simulink model "Model"  (R2024b)
settings: Solver=ode45  StartTime=0.0  StopTime=20  FixedStep=0.0005  MaxStep=InternalTs  RelTol=1e-3
InitFcn:
  | Design
values from neighbouring files (symbols this model uses):
  A = T \ A * T    [Design.m]
  Ao = A - L*C    [Design.m]
  B = T \ B    [Design.m]
  Bo = [B, L]    [Design.m]
  C = [1, 0, 0, 0]    [Design.m]
  D = 0    [Design.m]
  K = TmpK(2:end)    [Design.m]
  Ki = TmpK(1)    [Design.m]
  Nr = Nu + K * Nx    [Design.m]
  Ref = 50    [Design.m]
undefined symbols (not defined in the file or in its folder): DiscIntNeverNeededParam, InternalTs, RD, sens, t1
libraries: simulink_extras x6, simulink x2
settings Model: Creator=Banaan  LastModifiedBy=Banaan

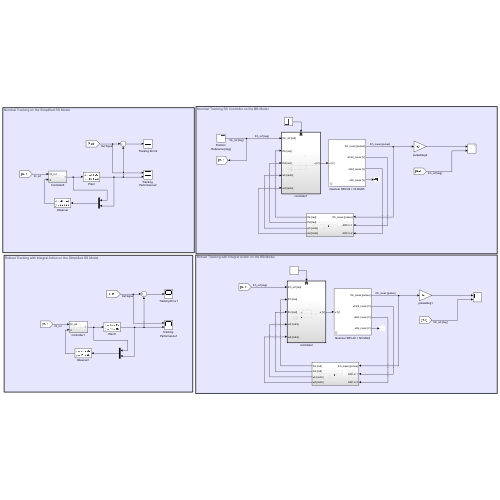
[thumbnail: Simulink's stored preview of the top-level diagram]
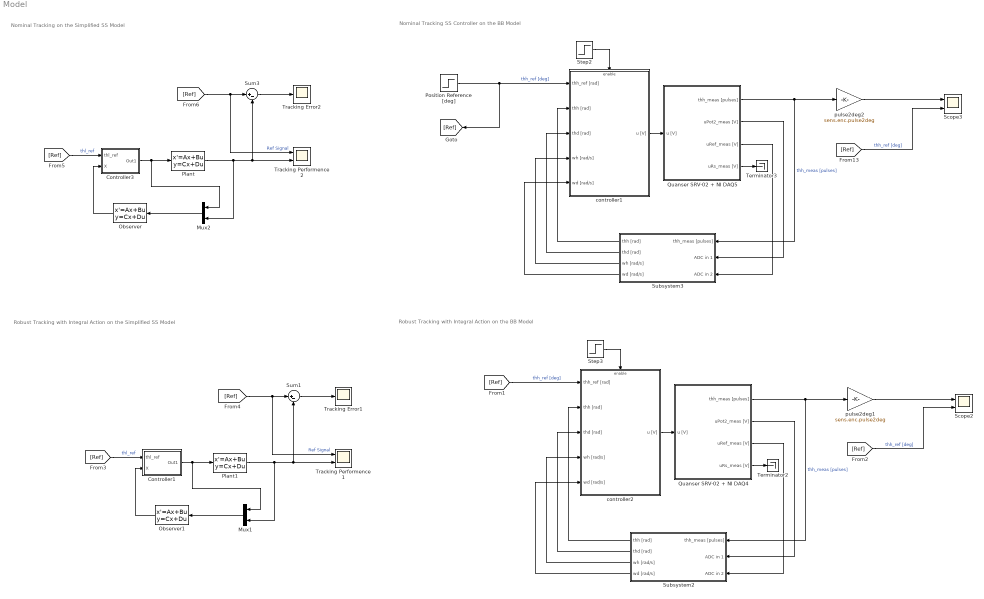
== system Model ==
  note: Robust Tracking with Integral Action on the BB Model
  note: Robust Tracking with Integral Action on the Simplified SS Model
  note: Nominal Tracking on the Simplified SS Model
  note: Nominal Tracking SS Controller on the BB Model
  Controller1 : Subsystem
  Controller3 : Subsystem
  Mux1 : Mux  Inputs=2
  Mux2 : Mux  Inputs=2
  Observer : StateSpace  A=Ao  B=Bo  C=eye(4)  D=zeros(4, 2)  InitialCondition=0
  Observer1 : StateSpace  A=Ao  B=Bo  C=eye(4)  D=zeros(4, 2)  InitialCondition=0
  Plant : StateSpace  A=A  B=B  C=C  D=D  InitialCondition=0
  Plant1 : StateSpace  A=A  B=B  C=C  D=D  InitialCondition=0
  Position Reference [deg] : Step  After=Ref  SampleTime=0
  Quanser SRV-02 + NI DAQ4 : Subsystem  mask(Quanser SRV-02 (with resonant load) + NI DAQ){Ts=0.001, fricType=Coulomb + viscous, lockShaft=off, beamInitPos=10}
      mask prompts: Ts "NI DAQ Sample Time:"; fricType "Friction model"; lockShaft "Lock motor shaft"; beamInitPos "Beam initial position [deg]:"
      mask help: Quanser SRV-02 (with resonant load) + NI DAQ model.
      mask init:
      | %%
      | % Riccardo Antonello (riccardo.antonello@unipd.it)
      | %
      | % April 28, 2020
      | %
      | % Dept. of Information Engineering, University of Padova
      | %
      | 
      | %%  Conversion gains
      | deg2rad = pi/180;                   %   [deg]   -> [rad]
      | rad2deg = 180/pi;                   %   [rad]   -> [deg]
      | 
      | 
      | %%  Sensors data
      | 
      | %   shunt resistor
      | sens.curr.Rs = 0.5;   
      | 
      | %   Hewlett-Packard HEDS-5540#A06 optical encoder
      | sens.enc.ppr = 500*4;                                                   %   pulses per rotation
      | sens.enc.pulse2deg = 360/sens.enc.ppr;                                  %   [pulses] -> [deg]
      | sens.enc.pulse2rad = 2*pi/sens.enc.ppr;                                 %   [pulses] -> [rad]
      | sens.enc.deg2pulse = sens.enc.ppr/360;                                  %   [deg] -> [pulses]
      | sens.enc.rad2pulse = sens.enc.ppr/2/pi;                                 %   [rad] -> [pulses]
      | 
      | %   potentiometer 2 (Spectrol 357-0-0-103) - installed on hub
      | sens.pot2.range.R      = 10e3;                                          %   ohmic value range 
      | sens.pot2.range.V      = 5;                                             %   voltage range
      | sens.pot2.range.th_deg = 340;                                           %   angle range [deg]
      | sens.pot2.range.th     = sens.pot2.range.th_deg * deg2rad;              %   angle range [rad]                           
      | sens.pot2.deg2V        = sens.pot2.range.V / sens.pot2.range.th_deg;    %   sensitivity [V/deg]
      | sens.pot2.rad2V        = sens.pot2.range.V / sens.pot2.range.th;        %   sensitivity [V/rad]
      | sens.pot2.V2deg        = 1/sens.pot2.deg2V;                             %   conversion gain [V] -> [deg]
      | sens.pot2.V2rad        = 1/sens.pot2.rad2V;                             %   conversion gain [V] -> [rad]
      | sens.pot2.noise.var    = 3.5e-7;                                        %   out noise variance [V^2]
      | 
      | 
      | %%  Data acquisition board (daq) data
      | 
      | %   NI PCI-6221 DAC data
      | daq.dac.bits = 16;                                  %   resolution (bits)
      | daq.dac.fs   = 10;                                  %   full scale 
      | daq.dac.q    = 2*daq.dac.fs/(2^daq.dac.bits-1);     %	quantization
      | 
      | %   NI PCI-6221 ADC data
      | daq.adc.bits = 16;                                  %   resolution (bits)
      | daq.adc.fs   = 10;                                  %   full scale (as set in SLDRT Analog Input block)
      | daq.adc.q    = 2*daq.adc.fs/(2^daq.adc.bits-1);     %   quantization   
      | 
      | 
      | %%  Set beam initial position
      | % SRV02Handle = find_system(gcb, ...
      | %     'LookUnderMasks', 'on', ...
      | %     'FindAll', 'on', ...
      | %     'FollowLinks', 'on', ...
      | %     'SearchDepth', '1', ...
      | %     'BlockType', 'ModelReference', ...
      | %     'Name', 'Quanser SRV-02');
      | %
      | % %get_param(SRV02Handle, 'InstanceParameters')
      | % InstanceParams = get_param(SRV02Handle, 'InstanceParameters');
      | % for k = 1:length(InstanceParams)
      | %     if strcmp(InstanceParams(k).Name, 'thb0')
      | %         if lockShaft
      | %             InstanceParams(k).Value = sprintf('%f', beamInitPos);
      | %         else
      | %             InstanceParams(k).Value = sprintf('%f', 0);    
      | %         end
      | %         set_param(SRV02Handle, 'InstanceParameters', InstanceParams);
      | %         break;
      | %     end
      | % end
      | 
      | if lockShaft
      |     thb0 = beamInitPos;
      | else
      |     thb0 = 0;    
      | end
      | 
      | 
      | %%  Mask initialization
      | if lockShaft
      |     
      |     %   find Inport handle
      |     InPortHandle = find_system(gcb, ...
      |         'LookUnderMasks', 'on', ...
      |         'FindAll', 'on', ...
      |         'FollowLinks', 'on', ...
      |         'SearchDepth', '1', ...
      |         'BlockType', 'Inport', ...
      |         'Name', 'u [V]');
      |     
      |     if ~isempty(InPortHandle)
      |     
      |         %   find DAC handle
      |         DACHandle = find_system(gcb, ...
      |             'LookUnderMasks', 'on', ...
      |             'FindAll', 'on', ...
      |             'FollowLinks', 'on', ...
      |             'SearchDepth', '1', ...
      |             'BlockType', 'SubSystem', ...
      |             'Name', 'DAC');  
      | 
      |         %   remove Inport output connection   
      |         InportConn = get_param(InPortHandle, 'PortConnectivity');
      |         delete_line(gcb, InportConn.Position);
      | 
      |         %   remove Inport block
      |         delete_block(InPortHandle);
      | 
      |         %   add Constant block
      |         ConstantHandle = add_block( ...
      |             'simulink/Sources/Constant', [gcb, '/u [V]'], ...
      |             'Position', [20   -37    50   -23], ...
      |             'Value', '0');
      | 
      |         %   connect Constant to DAC block
      |         DACPortHandles = get_param(DACHandle, 'PortHandles');
      |         ConstantPortHandles = get_param(ConstantHandle, 'PortHandles');
      |         add_line(gcb, ConstantPortHandles.Outport(1), DACPortHandles.Inport(1));
      |     
      |     end
      |     
      | else
      |     
      |     %   find Constant handle
      |     ConstantHandle = find_system(gcb, ...
      |         'LookUnderMasks', 'on', ...
      |         'FindAll', 'on', ...
      |         'FollowLinks', 'on', ...
      |         'SearchDepth', '1', ...
      |         'BlockType', 'Constant', ...
      |         'Name', 'u [V]');
      |     
      |     if ~isempty(ConstantHandle)
      |     
      |         %   find DAC handle
      |         DACHandle = find_system(gcb, ...
      |             'LookUnderMasks', 'on', ...
      |             'FindAll', 'on', ...
      |             'FollowLinks', 'on', ...
      |             'SearchDepth', '1', ...
      |             'BlockType', 'SubSystem', ...
      |             'Name', 'DAC');  
      |  
      |         %   remove Constant output connection   
      |         ConstantConn = get_param(ConstantHandle, 'PortConnectivity');
      |         delete_line(gcb, ConstantConn.Position);
      | 
      |         %   remove Inport block
      |         delete_block(ConstantHandle);   
      | 
      |         %   add Inport block
      |         InportHandle = add_block( ...
      |             'simulink/Sources/In1', [gcb, '/u [V]'], ...
      |             'Position', [20   -37    50   -23], ...
      |             'Port', '1');
      | 
      |         %   connect Constant to DAC block
      |         DACPortHandles = get_param(DACHandle, 'PortHandles');
      |         InportPortHandles = get_param(InportHandle, 'PortHandles');
      |         add_line(gcb, InportPortHandles.Outport(1), DACPortHandles.Inport(1));
      |     
      |      end
      |     
      | end
      mask Help:
      | Riccardo Antonello (antonello@dei.unipd.it)
      | 
      | April 28, 2020
      | 
      | Dept. of Information Engineering, University of Padova
      mask TypeOptions fricType: Coulomb + viscous | Karnopp
      mask Callback lockShaft:
      | %   get status of check box
      | lockShaft = get_param(gcb, 'lockShaft');
      | 
      | %   get current value of MaskVisibilities property
      | maskVisibilities = get_param(gcb, 'MaskVisibilities');
      | 
      | %   set visibility of the dialog box element
      | if strcmp(lockShaft, 'on')
      |     maskVisibilities{4} = 'on';
      | else
      |     maskVisibilities{4} = 'off';
      | end
      | 
      | % Set the 'MaskVisibilities' property for each parameter in mask
      | set_param( gcb, 'MaskVisibilities', maskVisibilities);
  Quanser SRV-02 + NI DAQ5 : Subsystem  mask(Quanser SRV-02 (with resonant load) + NI DAQ){Ts=0.001, fricType=Coulomb + viscous, lockShaft=off, beamInitPos=10}
      mask prompts: Ts "NI DAQ Sample Time:"; fricType "Friction model"; lockShaft "Lock motor shaft"; beamInitPos "Beam initial position [deg]:"
      mask help: Quanser SRV-02 (with resonant load) + NI DAQ model.
      mask init: same as Model/Quanser SRV-02 + NI DAQ4
      mask Help:
      | Riccardo Antonello (antonello@dei.unipd.it)
      | 
      | April 28, 2020
      | 
      | Dept. of Information Engineering, University of Padova
      mask TypeOptions fricType: Coulomb + viscous | Karnopp
      mask Callback lockShaft:
      | %   get status of check box
      | lockShaft = get_param(gcb, 'lockShaft');
      | 
      | %   get current value of MaskVisibilities property
      | maskVisibilities = get_param(gcb, 'MaskVisibilities');
      | 
      | %   set visibility of the dialog box element
      | if strcmp(lockShaft, 'on')
      |     maskVisibilities{4} = 'on';
      | else
      |     maskVisibilities{4} = 'off';
      | end
      | 
      | % Set the 'MaskVisibilities' property for each parameter in mask
      | set_param( gcb, 'MaskVisibilities', maskVisibilities);
  Scope2 : Scope  NumInputPorts=2
  Scope3 : Scope  NumInputPorts=2
  Step2 : Step  Time=t1 + 0.01  SampleTime=0
  Step3 : Step  Time=t1 + 0.01  SampleTime=0
  Subsystem2 : Subsystem
  Subsystem3 : Subsystem
  Sum1 : Sum  Inputs=|+-
  Sum3 : Sum  Inputs=|+-
  Terminator2 : Terminator
  Terminator3 : Terminator
  Tracking Performence1 : Scope  NumInputPorts=2
  Tracking Performence2 : Scope  NumInputPorts=2
  Tracking Error1 : Scope
  Tracking Error2 : Scope
  controller1 : Subsystem
  controller2 : Subsystem
  pulse2deg1 : Gain  Gain=sens.enc.pulse2deg
  pulse2deg2 : Gain  Gain=sens.enc.pulse2deg
  wires:
  [Ref] -> Tracking Performence2/1, Sum3/1  "Ref Signal"
  Sum3/1 -> Tracking Error2/1
  Plant/1 -> Tracking Performence2/2, Sum3/2, Mux2/2
  Mux2/1 -> Observer/1
  [Ref] -> Scope3/2  "thh_ref [deg]"
  pulse2deg2/1 -> Scope3/1
  Subsystem3/4(wd [rad/s]) -> controller1/5(wd [rad/s])
  Subsystem3/3(wh [rad/s]) -> controller1/4(wh [rad/s])
  Subsystem3/2(thd [rad]) -> controller1/3(thd [rad])
  Subsystem3/1(thh [rad]) -> controller1/2(thh [rad])
  Quanser SRV-02 + NI DAQ5/3(uRef_meas [V]) -> Subsystem3/3(ADC in 2)
  Quanser SRV-02 + NI DAQ5/2(uPot2_meas [V]) -> Subsystem3/2(ADC in 1)
  Quanser SRV-02 + NI DAQ5/1(thh_meas [pulses]) -> Subsystem3/1(thh_meas [pulses]), pulse2deg2/1  "thh_meas [pulses]"
  controller1/1(u [V]) -> Quanser SRV-02 + NI DAQ5/1(u [V])
  Step2/1 -> controller1/Enable
  Quanser SRV-02 + NI DAQ5/4(uRs_meas [V]) -> Terminator3/1
  Position Reference [deg]/1 -> controller1/1(thh_ref [rad]), [Ref]  "thh_ref [deg]"
  Controller3/1(Out1) -> Plant/1, Mux2/1
  [Ref] -> Controller3/1(thl_ref)  "thl_ref"
  Observer/1 -> Controller3/2(X)
  [Ref] -> controller2/1(thh_ref [rad])  "thh_ref [deg]"
  Quanser SRV-02 + NI DAQ4/4(uRs_meas [V]) -> Terminator2/1
  Step3/1 -> controller2/Enable
  controller2/1(u [V]) -> Quanser SRV-02 + NI DAQ4/1(u [V])
  Quanser SRV-02 + NI DAQ4/1(thh_meas [pulses]) -> pulse2deg1/1, Subsystem2/1(thh_meas [pulses])  "thh_meas [pulses]"
  Quanser SRV-02 + NI DAQ4/2(uPot2_meas [V]) -> Subsystem2/2(ADC in 1)
  Quanser SRV-02 + NI DAQ4/3(uRef_meas [V]) -> Subsystem2/3(ADC in 2)
  Subsystem2/1(thh [rad]) -> controller2/2(thh [rad])
  Subsystem2/2(thd [rad]) -> controller2/3(thd [rad])
  Subsystem2/3(wh [rad/s]) -> controller2/4(wh [rad/s])
  Subsystem2/4(wd [rad/s]) -> controller2/5(wd [rad/s])
  pulse2deg1/1 -> Scope2/1
  [Ref] -> Scope2/2  "thh_ref [deg]"
  Observer1/1 -> Controller1/2(X)
  [Ref] -> Controller1/1(thl_ref)  "thl_ref"
  Controller1/1(Out1) -> Mux1/1, Plant1/1
  Mux1/1 -> Observer1/1
  Plant1/1 -> Mux1/2, Sum1/2, Tracking Performence1/2
  Sum1/1 -> Tracking Error1/1
  [Ref] -> Sum1/1, Tracking Performence1/1  "Ref Signal"

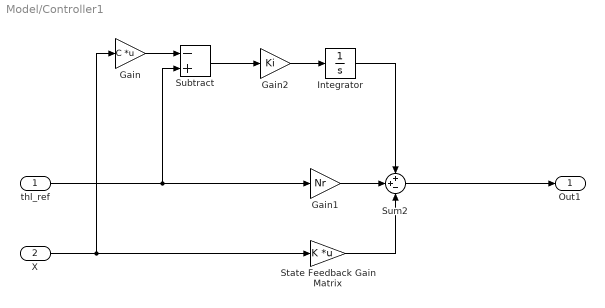
== system Model/Controller1 ==
  thl_ref : Inport
  X : Inport  Port=2
  Gain : Gain  Gain=C  Multiplication=Matrix(K*u)
  Gain1 : Gain  Gain=Nr
  Gain2 : Gain  Gain=Ki
  Integrator : Integrator
  State Feedback Gain Matrix : Gain  Gain=K  Multiplication=Matrix(K*u)
  Subtract : Sum  Inputs=-+
  Sum2 : Sum  Inputs=++-
  Out1 : Outport
  wires:
  Sum2/1 -> Out1/1
  X/1 -> Gain/1, State Feedback Gain Matrix/1
  Gain1/1 -> Sum2/2
  State Feedback Gain Matrix/1 -> Sum2/3
  Gain/1 -> Subtract/1
  thl_ref/1 -> Gain1/1, Subtract/2
  Subtract/1 -> Gain2/1
  Gain2/1 -> Integrator/1
  Integrator/1 -> Sum2/1

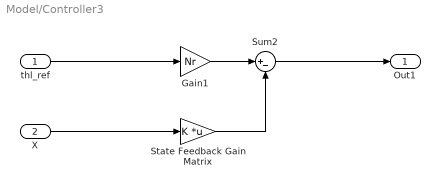
== system Model/Controller3 ==
  thl_ref : Inport
  X : Inport  Port=2
  Gain1 : Gain  Gain=Nr
  State Feedback Gain Matrix : Gain  Gain=K  Multiplication=Matrix(K*u)
  Sum2 : Sum  Inputs=|+-
  Out1 : Outport
  wires:
  State Feedback Gain Matrix/1 -> Sum2/2
  Gain1/1 -> Sum2/1
  X/1 -> State Feedback Gain Matrix/1
  thl_ref/1 -> Gain1/1
  Sum2/1 -> Out1/1

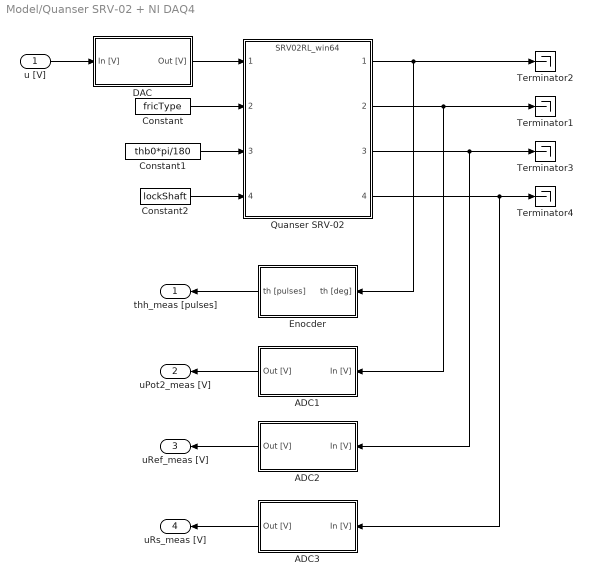
== system Model/Quanser SRV-02 + NI DAQ4 ==
  u [V] : Inport
  ADC1 : Subsystem
  ADC2 : Subsystem
  ADC3 : Subsystem
  Constant : Constant  Value=fricType
  Constant1 : Constant  Value=thb0*pi/180  SampleTime=Inf
  Constant2 : Constant  Value=lockShaft  SampleTime=Inf
  DAC : Subsystem
  Enocder : Subsystem
  Quanser SRV-02 : ModelReference  ModelNameDialog=SRV02RL_win64.slxp  ModelReferenceVersion=1.76  CopyOfModelProtected=on
  Terminator{1..4} (4 alike) : Terminator
  thh_meas [pulses] : Outport
  uPot2_meas [V] : Outport  Port=2
  uRef_meas [V] : Outport  Port=3
  uRs_meas [V] : Outport  Port=4
  wires:
  u [V]/1 -> DAC/1(In [V])
  ADC2/1(Out [V]) -> uRef_meas [V]/1
  Quanser SRV-02/4 -> Terminator4/1, ADC3/1(In [V])
  Constant2/1 -> Quanser SRV-02/4
  Constant1/1 -> Quanser SRV-02/3
  ADC1/1(Out [V]) -> uPot2_meas [V]/1
  Quanser SRV-02/3 -> Terminator3/1, ADC2/1(In [V])
  Constant/1 -> Quanser SRV-02/2
  Quanser SRV-02/1 -> Enocder/1(th [deg]), Terminator2/1
  Quanser SRV-02/2 -> Terminator1/1, ADC1/1(In [V])
  DAC/1(Out [V]) -> Quanser SRV-02/1
  ADC3/1(Out [V]) -> uRs_meas [V]/1
  Enocder/1(th [pulses]) -> thh_meas [pulses]/1

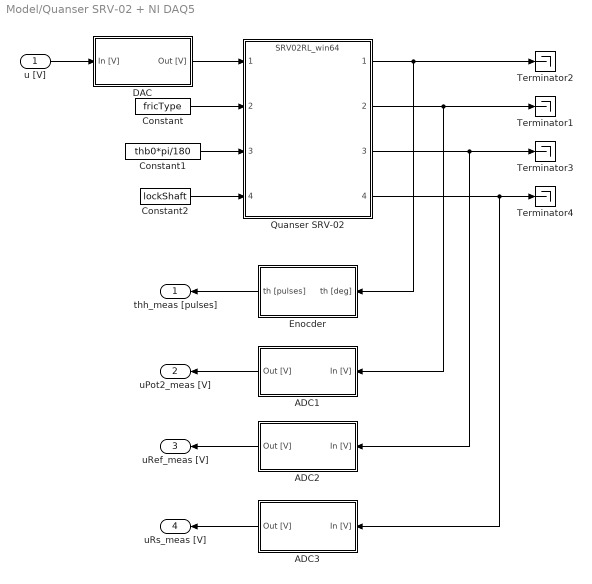
== system Model/Quanser SRV-02 + NI DAQ5 ==
  u [V] : Inport
  ADC1 : Subsystem
  ADC2 : Subsystem
  ADC3 : Subsystem
  Constant : Constant  Value=fricType
  Constant1 : Constant  Value=thb0*pi/180  SampleTime=Inf
  Constant2 : Constant  Value=lockShaft  SampleTime=Inf
  DAC : Subsystem
  Enocder : Subsystem
  Quanser SRV-02 : ModelReference  ModelNameDialog=SRV02RL_win64.slxp  ModelReferenceVersion=1.76  CopyOfModelProtected=on
  Terminator{1..4} (4 alike) : Terminator
  thh_meas [pulses] : Outport
  uPot2_meas [V] : Outport  Port=2
  uRef_meas [V] : Outport  Port=3
  uRs_meas [V] : Outport  Port=4
  wires:
  Enocder/1(th [pulses]) -> thh_meas [pulses]/1
  ADC3/1(Out [V]) -> uRs_meas [V]/1
  DAC/1(Out [V]) -> Quanser SRV-02/1
  Quanser SRV-02/2 -> ADC1/1(In [V]), Terminator1/1
  Quanser SRV-02/1 -> Terminator2/1, Enocder/1(th [deg])
  Constant/1 -> Quanser SRV-02/2
  Quanser SRV-02/3 -> ADC2/1(In [V]), Terminator3/1
  ADC1/1(Out [V]) -> uPot2_meas [V]/1
  Constant1/1 -> Quanser SRV-02/3
  Constant2/1 -> Quanser SRV-02/4
  Quanser SRV-02/4 -> ADC3/1(In [V]), Terminator4/1
  ADC2/1(Out [V]) -> uRef_meas [V]/1
  u [V]/1 -> DAC/1(In [V])

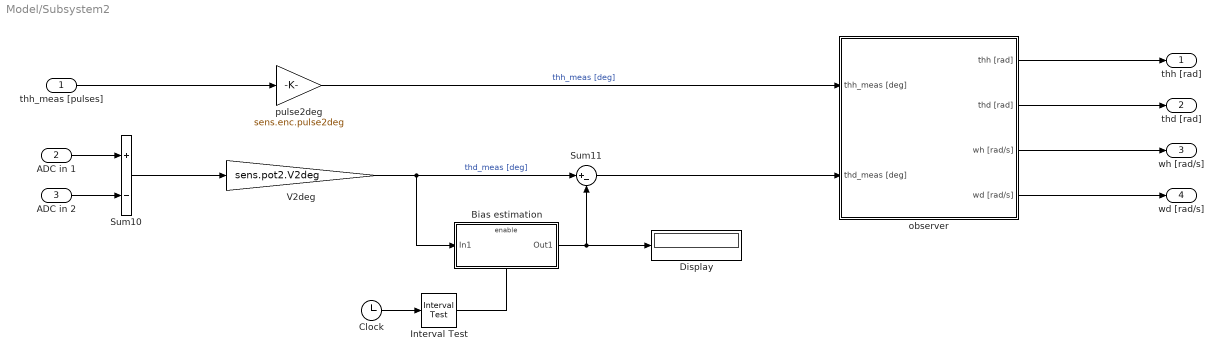
== system Model/Subsystem2 ==
  thh_meas [pulses] : Inport
  ADC in 1 : Inport  Port=2
  ADC in 2 : Inport  Port=3
  Bias estimation : Subsystem
  Clock : Clock
  Display : Display
  Interval Test : simulink/Logic and Bit Operations/Interval Test  IntervalClosedRight=on  uplimit=0.7  IntervalClosedLeft=on  lowlimit=0.2  OutDataTypeStr=boolean
  Sum10 : Sum  Inputs=+-
  Sum11 : Sum  Inputs=|+-
  V2deg : Gain  Gain=sens.pot2.V2deg
  observer : Subsystem
  pulse2deg : Gain  Gain=sens.enc.pulse2deg
  thh [rad] : Outport
  thd [rad] : Outport  Port=2
  wh [rad/s] : Outport  Port=3
  wd [rad/s] : Outport  Port=4
  wires:
  Bias estimation/1(Out1) -> Display/1, Sum11/2
  observer/1(thh [rad]) -> thh [rad]/1
  Interval Test/1 -> Bias estimation/Enable
  Sum10/1 -> V2deg/1
  thh_meas [pulses]/1 -> pulse2deg/1
  observer/4(wd [rad/s]) -> wd [rad/s]/1
  pulse2deg/1 -> observer/1(thh_meas [deg])  "thh_meas [deg]"
  ADC in 2/1 -> Sum10/2
  V2deg/1 -> Sum11/1, Bias estimation/1(In1)  "thd_meas [deg]"
  Sum11/1 -> observer/2(thd_meas [deg])
  Clock/1 -> Interval Test/1
  observer/2(thd [rad]) -> thd [rad]/1
  ADC in 1/1 -> Sum10/1
  observer/3(wh [rad/s]) -> wh [rad/s]/1

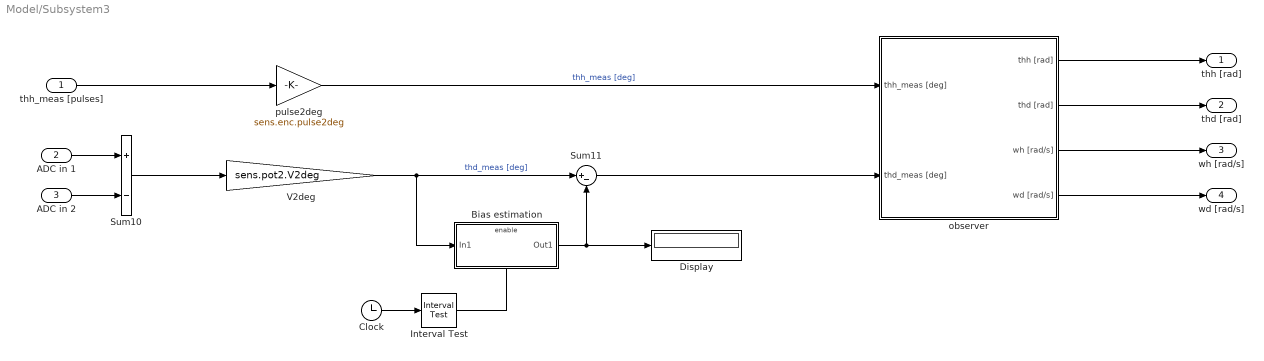
== system Model/Subsystem3 ==
  thh_meas [pulses] : Inport
  ADC in 1 : Inport  Port=2
  ADC in 2 : Inport  Port=3
  Bias estimation : Subsystem
  Clock : Clock
  Display : Display
  Interval Test : simulink/Logic and Bit Operations/Interval Test  IntervalClosedRight=on  uplimit=0.7  IntervalClosedLeft=on  lowlimit=0.2  OutDataTypeStr=boolean
  Sum10 : Sum  Inputs=+-
  Sum11 : Sum  Inputs=|+-
  V2deg : Gain  Gain=sens.pot2.V2deg
  observer : Subsystem
  pulse2deg : Gain  Gain=sens.enc.pulse2deg
  thh [rad] : Outport
  thd [rad] : Outport  Port=2
  wh [rad/s] : Outport  Port=3
  wd [rad/s] : Outport  Port=4
  wires:
  observer/3(wh [rad/s]) -> wh [rad/s]/1
  ADC in 1/1 -> Sum10/1
  observer/2(thd [rad]) -> thd [rad]/1
  Clock/1 -> Interval Test/1
  Sum11/1 -> observer/2(thd_meas [deg])
  V2deg/1 -> Bias estimation/1(In1), Sum11/1  "thd_meas [deg]"
  ADC in 2/1 -> Sum10/2
  pulse2deg/1 -> observer/1(thh_meas [deg])  "thh_meas [deg]"
  observer/4(wd [rad/s]) -> wd [rad/s]/1
  thh_meas [pulses]/1 -> pulse2deg/1
  Sum10/1 -> V2deg/1
  Interval Test/1 -> Bias estimation/Enable
  observer/1(thh [rad]) -> thh [rad]/1
  Bias estimation/1(Out1) -> Sum11/2, Display/1

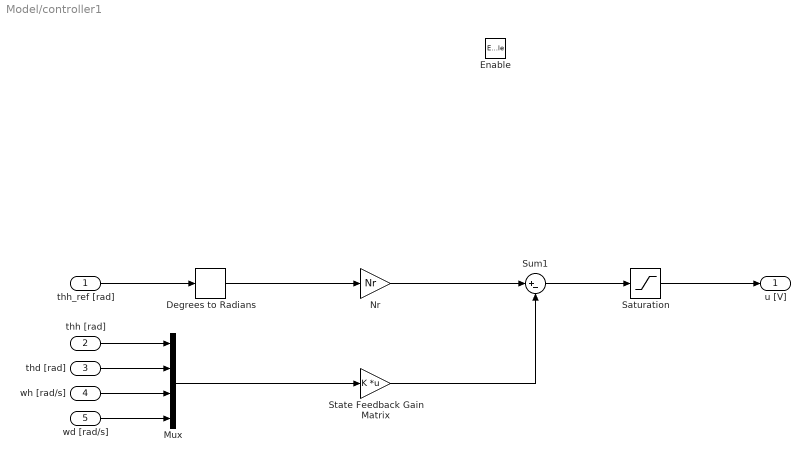
== system Model/controller1 ==
  thh_ref [rad] : Inport
  thh [rad] : Inport  Port=2
  thd [rad] : Inport  Port=3
  wh [rad/s] : Inport  Port=4
  wd [rad/s] : Inport  Port=5
  Enable : EnablePort
  Degrees to Radians : simulink_extras/Transformations/Degrees to Radians
  Mux : Mux
  Nr : Gain  Gain=Nr
  Saturation : Saturate  UpperLimit=10  LowerLimit=-10
  State Feedback Gain Matrix : Gain  Gain=K  Multiplication=Matrix(K*u)
  Sum1 : Sum  Inputs=|+-
  u [V] : Outport
  wires:
  Degrees to Radians/1 -> Nr/1
  Saturation/1 -> u [V]/1
  Mux/1 -> State Feedback Gain Matrix/1
  Nr/1 -> Sum1/1
  Sum1/1 -> Saturation/1
  wd [rad/s]/1 -> Mux/4
  wh [rad/s]/1 -> Mux/3
  thd [rad]/1 -> Mux/2
  thh [rad]/1 -> Mux/1
  State Feedback Gain Matrix/1 -> Sum1/2
  thh_ref [rad]/1 -> Degrees to Radians/1

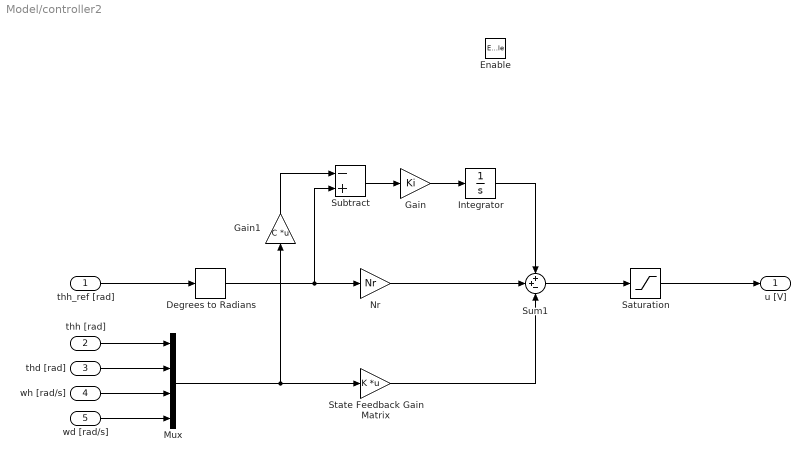
== system Model/controller2 ==
  thh_ref [rad] : Inport
  thh [rad] : Inport  Port=2
  thd [rad] : Inport  Port=3
  wh [rad/s] : Inport  Port=4
  wd [rad/s] : Inport  Port=5
  Enable : EnablePort
  Degrees to Radians : simulink_extras/Transformations/Degrees to Radians
  Gain : Gain  Gain=Ki
  Gain1 : Gain  Gain=C  Multiplication=Matrix(K*u)
  Integrator : Integrator
  Mux : Mux
  Nr : Gain  Gain=Nr
  Saturation : Saturate  UpperLimit=10  LowerLimit=-10
  State Feedback Gain Matrix : Gain  Gain=K  Multiplication=Matrix(K*u)
  Subtract : Sum  Inputs=-+
  Sum1 : Sum  Inputs=++-
  u [V] : Outport
  wires:
  thh_ref [rad]/1 -> Degrees to Radians/1
  State Feedback Gain Matrix/1 -> Sum1/3
  thh [rad]/1 -> Mux/1
  thd [rad]/1 -> Mux/2
  wh [rad/s]/1 -> Mux/3
  wd [rad/s]/1 -> Mux/4
  Sum1/1 -> Saturation/1
  Nr/1 -> Sum1/2
  Mux/1 -> State Feedback Gain Matrix/1, Gain1/1
  Saturation/1 -> u [V]/1
  Degrees to Radians/1 -> Subtract/2, Nr/1
  Gain/1 -> Integrator/1
  Subtract/1 -> Gain/1
  Integrator/1 -> Sum1/1
  Gain1/1 -> Subtract/1

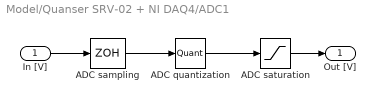
== system Model/Quanser SRV-02 + NI DAQ4/ADC1 ==
  In [V] : Inport
  ADC quantization : Quantizer  QuantizationInterval=daq.adc.q
  ADC sampling : ZeroOrderHold  SampleTime=Ts
  ADC saturation : Saturate  UpperLimit=daq.adc.fs  LowerLimit=-daq.adc.fs
  Out [V] : Outport
  wires:
  ADC quantization/1 -> ADC saturation/1
  In [V]/1 -> ADC sampling/1
  ADC sampling/1 -> ADC quantization/1
  ADC saturation/1 -> Out [V]/1

== system Model/Quanser SRV-02 + NI DAQ4/ADC2 ==
  In [V] : Inport
  ADC quantization : Quantizer  QuantizationInterval=daq.adc.q
  ADC sampling : ZeroOrderHold  SampleTime=Ts
  ADC saturation : Saturate  UpperLimit=daq.adc.fs  LowerLimit=-daq.adc.fs
  Out [V] : Outport
  wires:
  ADC saturation/1 -> Out [V]/1
  ADC sampling/1 -> ADC quantization/1
  In [V]/1 -> ADC sampling/1
  ADC quantization/1 -> ADC saturation/1

== system Model/Quanser SRV-02 + NI DAQ4/ADC3 ==
  In [V] : Inport
  Quantizer : Quantizer  QuantizationInterval=daq.adc.q
  Saturation : Saturate  UpperLimit=daq.adc.fs  LowerLimit=-daq.adc.fs
  Zero-Order Hold : ZeroOrderHold  SampleTime=Ts
  Out [V] : Outport
  wires:
  Zero-Order Hold/1 -> Quantizer/1
  Quantizer/1 -> Saturation/1
  In [V]/1 -> Zero-Order Hold/1
  Saturation/1 -> Out [V]/1

== system Model/Quanser SRV-02 + NI DAQ4/DAC ==
  In [V] : Inport
  Quantizer : Quantizer  QuantizationInterval=daq.dac.q
  Saturation : Saturate  UpperLimit=daq.dac.fs  LowerLimit=-daq.dac.fs
  Zero-Order Hold : ZeroOrderHold  SampleTime=Ts
  Out [V] : Outport
  wires:
  Saturation/1 -> Out [V]/1
  Zero-Order Hold/1 -> Quantizer/1
  In [V]/1 -> Zero-Order Hold/1
  Quantizer/1 -> Saturation/1

== system Model/Quanser SRV-02 + NI DAQ4/Enocder ==
  th [deg] : Inport
  Quantizer : Quantizer  QuantizationInterval=sens.enc.pulse2deg
  Zero-Order Hold : ZeroOrderHold  SampleTime=Ts
  deg2pulse : Gain  Gain=sens.enc.deg2pulse
  th [pulses] : Outport
  wires:
  deg2pulse/1 -> th [pulses]/1
  Zero-Order Hold/1 -> Quantizer/1
  th [deg]/1 -> Zero-Order Hold/1
  Quantizer/1 -> deg2pulse/1

== system Model/Quanser SRV-02 + NI DAQ5/ADC1 ==
  In [V] : Inport
  ADC quantization : Quantizer  QuantizationInterval=daq.adc.q
  ADC sampling : ZeroOrderHold  SampleTime=Ts
  ADC saturation : Saturate  UpperLimit=daq.adc.fs  LowerLimit=-daq.adc.fs
  Out [V] : Outport
  wires:
  ADC saturation/1 -> Out [V]/1
  ADC sampling/1 -> ADC quantization/1
  In [V]/1 -> ADC sampling/1
  ADC quantization/1 -> ADC saturation/1

== system Model/Quanser SRV-02 + NI DAQ5/ADC2 ==
  In [V] : Inport
  ADC quantization : Quantizer  QuantizationInterval=daq.adc.q
  ADC sampling : ZeroOrderHold  SampleTime=Ts
  ADC saturation : Saturate  UpperLimit=daq.adc.fs  LowerLimit=-daq.adc.fs
  Out [V] : Outport
  wires:
  ADC quantization/1 -> ADC saturation/1
  In [V]/1 -> ADC sampling/1
  ADC sampling/1 -> ADC quantization/1
  ADC saturation/1 -> Out [V]/1

== system Model/Quanser SRV-02 + NI DAQ5/ADC3 ==
  In [V] : Inport
  Quantizer : Quantizer  QuantizationInterval=daq.adc.q
  Saturation : Saturate  UpperLimit=daq.adc.fs  LowerLimit=-daq.adc.fs
  Zero-Order Hold : ZeroOrderHold  SampleTime=Ts
  Out [V] : Outport
  wires:
  Saturation/1 -> Out [V]/1
  In [V]/1 -> Zero-Order Hold/1
  Quantizer/1 -> Saturation/1
  Zero-Order Hold/1 -> Quantizer/1

== system Model/Quanser SRV-02 + NI DAQ5/DAC ==
  In [V] : Inport
  Quantizer : Quantizer  QuantizationInterval=daq.dac.q
  Saturation : Saturate  UpperLimit=daq.dac.fs  LowerLimit=-daq.dac.fs
  Zero-Order Hold : ZeroOrderHold  SampleTime=Ts
  Out [V] : Outport
  wires:
  Quantizer/1 -> Saturation/1
  In [V]/1 -> Zero-Order Hold/1
  Zero-Order Hold/1 -> Quantizer/1
  Saturation/1 -> Out [V]/1

== system Model/Quanser SRV-02 + NI DAQ5/Enocder ==
  th [deg] : Inport
  Quantizer : Quantizer  QuantizationInterval=sens.enc.pulse2deg
  Zero-Order Hold : ZeroOrderHold  SampleTime=Ts
  deg2pulse : Gain  Gain=sens.enc.deg2pulse
  th [pulses] : Outport
  wires:
  Quantizer/1 -> deg2pulse/1
  th [deg]/1 -> Zero-Order Hold/1
  Zero-Order Hold/1 -> Quantizer/1
  deg2pulse/1 -> th [pulses]/1

== system Model/Subsystem2/Bias estimation ==
  In1 : Inport
  Enable : EnablePort
  Discrete-Time Integrator : DiscreteIntegrator  gainval=BiasIntegratorGain  SampleTime=InternalTs  ICPrevOutput=DiscIntNeverNeededParam  ICPrevScaledInput=DiscIntNeverNeededParam
  Out1 : Outport
  wires:
  In1/1 -> Discrete-Time Integrator/1
  Discrete-Time Integrator/1 -> Out1/1

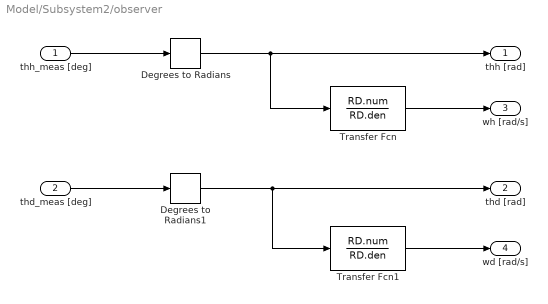
== system Model/Subsystem2/observer ==
  thh_meas [deg] : Inport
  thd_meas [deg] : Inport  Port=2
  Degrees to Radians : simulink_extras/Transformations/Degrees to Radians
  Degrees to Radians1 : simulink_extras/Transformations/Degrees to Radians
  Transfer Fcn : TransferFcn  Numerator=RD.num  Denominator=RD.den
  Transfer Fcn1 : TransferFcn  Numerator=RD.num  Denominator=RD.den
  thh [rad] : Outport
  thd [rad] : Outport  Port=2
  wh [rad/s] : Outport  Port=3
  wd [rad/s] : Outport  Port=4
  wires:
  thh_meas [deg]/1 -> Degrees to Radians/1
  thd_meas [deg]/1 -> Degrees to Radians1/1
  Transfer Fcn/1 -> wh [rad/s]/1
  Degrees to Radians1/1 -> Transfer Fcn1/1, thd [rad]/1
  Degrees to Radians/1 -> Transfer Fcn/1, thh [rad]/1
  Transfer Fcn1/1 -> wd [rad/s]/1

== system Model/Subsystem3/Bias estimation ==
  In1 : Inport
  Enable : EnablePort
  Discrete-Time Integrator : DiscreteIntegrator  gainval=BiasIntegratorGain  SampleTime=InternalTs  ICPrevOutput=DiscIntNeverNeededParam  ICPrevScaledInput=DiscIntNeverNeededParam
  Out1 : Outport
  wires:
  Discrete-Time Integrator/1 -> Out1/1
  In1/1 -> Discrete-Time Integrator/1

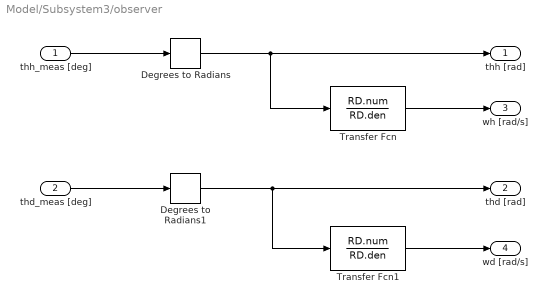
== system Model/Subsystem3/observer ==
  thh_meas [deg] : Inport
  thd_meas [deg] : Inport  Port=2
  Degrees to Radians : simulink_extras/Transformations/Degrees to Radians
  Degrees to Radians1 : simulink_extras/Transformations/Degrees to Radians
  Transfer Fcn : TransferFcn  Numerator=RD.num  Denominator=RD.den
  Transfer Fcn1 : TransferFcn  Numerator=RD.num  Denominator=RD.den
  thh [rad] : Outport
  thd [rad] : Outport  Port=2
  wh [rad/s] : Outport  Port=3
  wd [rad/s] : Outport  Port=4
  wires:
  Transfer Fcn1/1 -> wd [rad/s]/1
  Degrees to Radians/1 -> thh [rad]/1, Transfer Fcn/1
  Degrees to Radians1/1 -> thd [rad]/1, Transfer Fcn1/1
  Transfer Fcn/1 -> wh [rad/s]/1
  thd_meas [deg]/1 -> Degrees to Radians1/1
  thh_meas [deg]/1 -> Degrees to Radians/1
